simulink model "TCS_FrontAxle_Model"  (R2026a)
settings: Solver=ode4  StopTime=5  FixedStep=0.005
model workspace (MAT data in the model file):
  IntegralMax = 500
  IntegralMin = 0
  Ki = 200
  Kp = 800
  R_wheel = 0.25
  Tcorr_min_val = -500
  deadband = 0.02
  lambda_target = 0.1
  vx_min = 0.5
libraries: simulink x1
settings Model: Creator=liurui  LastModifiedBy=liurui

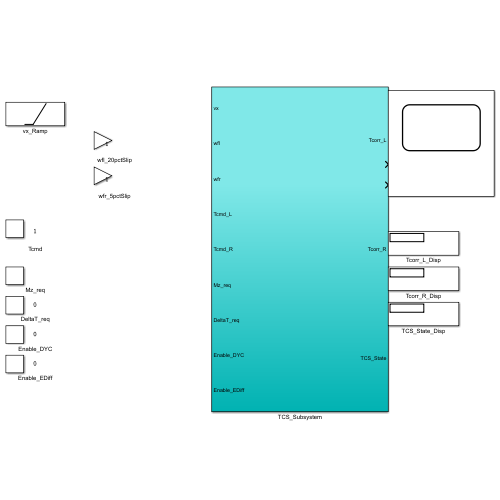
[thumbnail: Simulink's stored preview of the top-level diagram]
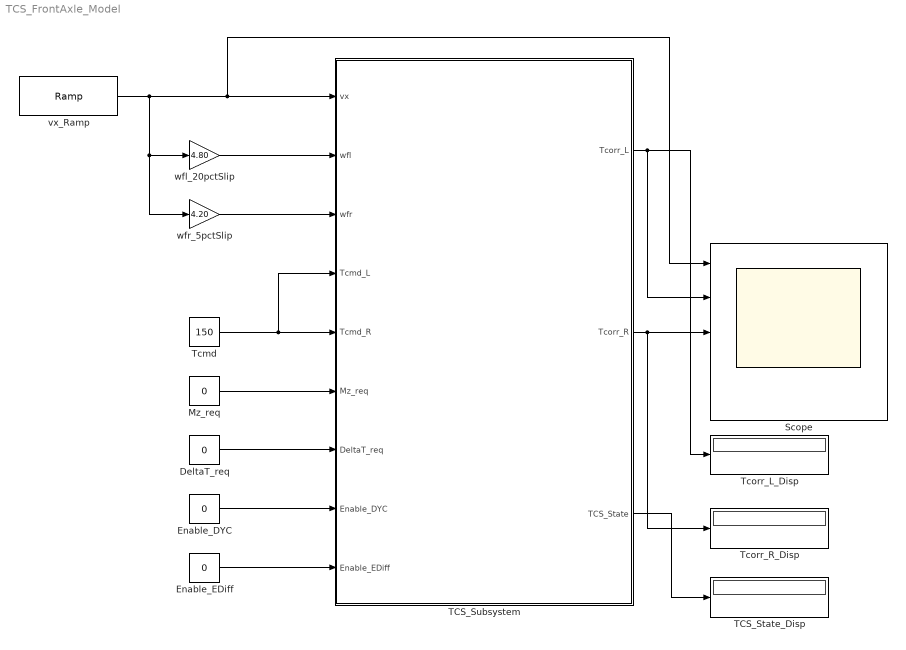
== system TCS_FrontAxle_Model ==
  DeltaT_req : Constant  Value=0
  Enable_DYC : Constant  Value=0
  Enable_EDiff : Constant  Value=0
  Mz_req : Constant  Value=0
  Scope : Scope  NumInputPorts=5
  TCS_State_Disp : Display
  TCS_Subsystem : Subsystem
  Tcmd : Constant  Value=150
  Tcorr_L_Disp : Display
  Tcorr_R_Disp : Display
  vx_Ramp : simulink/Sources/Ramp  slope=5  start=0.2  InitialOutput=0.1
  wfl_20pctSlip : Gain  Gain=4.80
  wfr_5pctSlip : Gain  Gain=4.20
  wires:
  vx_Ramp/1 -> wfl_20pctSlip/1, wfr_5pctSlip/1, TCS_Subsystem/1(vx), Scope/1
  Mz_req/1 -> TCS_Subsystem/6(Mz_req)
  Tcmd/1 -> TCS_Subsystem/4(Tcmd_L), TCS_Subsystem/5(Tcmd_R)
  wfr_5pctSlip/1 -> TCS_Subsystem/3(wfr)
  wfl_20pctSlip/1 -> TCS_Subsystem/2(wfl)
  Enable_EDiff/1 -> TCS_Subsystem/9(Enable_EDiff)
  Enable_DYC/1 -> TCS_Subsystem/8(Enable_DYC)
  TCS_Subsystem/2(Tcorr_R) -> Scope/3, Tcorr_R_Disp/1
  DeltaT_req/1 -> TCS_Subsystem/7(DeltaT_req)
  TCS_Subsystem/1(Tcorr_L) -> Scope/2, Tcorr_L_Disp/1
  TCS_Subsystem/3(TCS_State) -> TCS_State_Disp/1

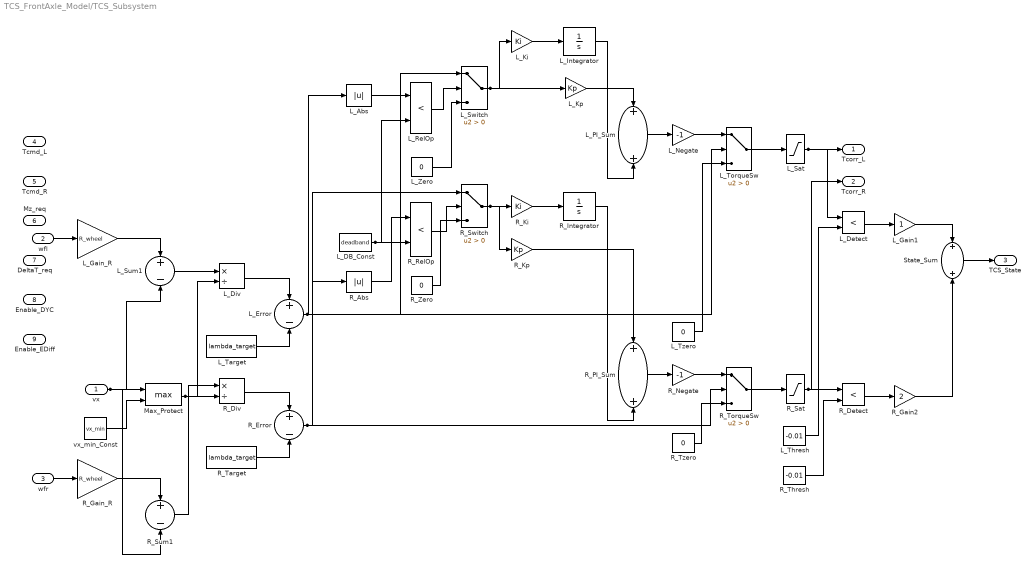
== system TCS_FrontAxle_Model/TCS_Subsystem ==
  vx : Inport
  wfl : Inport  Port=2
  wfr : Inport  Port=3
  Tcmd_L : Inport  Port=4
  Tcmd_R : Inport  Port=5
  Mz_req : Inport  Port=6
  DeltaT_req : Inport  Port=7
  Enable_DYC : Inport  Port=8
  Enable_EDiff : Inport  Port=9
  L_Abs : Abs  SaturateOnIntegerOverflow=off
  L_DB_Const : Constant  Value=deadband
  L_Detect : RelationalOperator  Operator=<  OutDataTypeStr=boolean  RndMeth=Simplest  InputSameDT=off
  L_Div : Product  Inputs=*/
  L_Error : Sum  Inputs=+-
  L_Gain1 : Gain
  L_Gain_R : Gain  Gain=R_wheel
  L_Integrator : Integrator  UpperSaturationLimit=IntegralMax  LowerSaturationLimit=IntegralMin
  L_Ki : Gain  Gain=Ki
  L_Kp : Gain  Gain=Kp
  L_Negate : Gain  Gain=-1
  L_PI_Sum : Sum
  L_RelOp : RelationalOperator  Operator=<  OutDataTypeStr=boolean  RndMeth=Simplest  InputSameDT=off
  L_Sat : Saturate  UpperLimit=0  LowerLimit=Tcorr_min_val
  L_Sum1 : Sum  Inputs=+-
  L_Switch : Switch  Criteria=u2 > Threshold  SaturateOnIntegerOverflow=off  InputSameDT=off
  L_Target : Constant  Value=lambda_target
  L_Thresh : Constant  Value=-0.01
  L_TorqueSw : Switch  Criteria=u2 > Threshold  SaturateOnIntegerOverflow=off  InputSameDT=off
  L_Tzero : Constant  Value=0
  L_Zero : Constant  Value=0
  Max_Protect : MinMax  Function=max  Inputs=2
  R_Abs : Abs  SaturateOnIntegerOverflow=off
  R_Detect : RelationalOperator  Operator=<  OutDataTypeStr=boolean  RndMeth=Simplest  InputSameDT=off
  R_Div : Product  Inputs=*/
  R_Error : Sum  Inputs=+-
  R_Gain2 : Gain  Gain=2
  R_Gain_R : Gain  Gain=R_wheel
  R_Integrator : Integrator  UpperSaturationLimit=IntegralMax  LowerSaturationLimit=IntegralMin
  R_Ki : Gain  Gain=Ki
  R_Kp : Gain  Gain=Kp
  R_Negate : Gain  Gain=-1
  R_PI_Sum : Sum
  R_RelOp : RelationalOperator  Operator=<  OutDataTypeStr=boolean  RndMeth=Simplest  InputSameDT=off
  R_Sat : Saturate  UpperLimit=0  LowerLimit=Tcorr_min_val
  R_Sum1 : Sum  Inputs=+-
  R_Switch : Switch  Criteria=u2 > Threshold  SaturateOnIntegerOverflow=off  InputSameDT=off
  R_Target : Constant  Value=lambda_target
  R_Thresh : Constant  Value=-0.01
  R_TorqueSw : Switch  Criteria=u2 > Threshold  SaturateOnIntegerOverflow=off  InputSameDT=off
  R_Tzero : Constant  Value=0
  R_Zero : Constant  Value=0
  State_Sum : Sum
  vx_min_Const : Constant  Value=vx_min
  Tcorr_L : Outport
  Tcorr_R : Outport  Port=2
  TCS_State : Outport  Port=3
  wires:
  wfr/1 -> R_Gain_R/1
  vx/1 -> R_Sum1/2, L_Sum1/2, Max_Protect/1
  wfl/1 -> L_Gain_R/1
  L_Ki/1 -> L_Integrator/1
  R_Switch/1 -> R_Kp/1, R_Ki/1
  L_Gain_R/1 -> L_Sum1/1
  vx_min_Const/1 -> Max_Protect/2
  Max_Protect/1 -> L_Div/2, R_Div/2
  R_Gain_R/1 -> R_Sum1/1
  L_Div/1 -> L_Error/1
  L_Sum1/1 -> L_Div/1
  R_Sum1/1 -> R_Div/1
  L_Negate/1 -> L_TorqueSw/1
  L_PI_Sum/1 -> L_Negate/1
  L_Target/1 -> L_Error/2
  R_Div/1 -> R_Error/1
  R_Target/1 -> R_Error/2
  L_Error/1 -> L_TorqueSw/2, L_Abs/1, L_Switch/1
  L_DB_Const/1 -> L_RelOp/2, R_RelOp/2
  R_Error/1 -> R_TorqueSw/2, R_Switch/1, R_Abs/1
  L_Abs/1 -> L_RelOp/1
  R_Abs/1 -> R_RelOp/1
  L_RelOp/1 -> L_Switch/2
  L_Zero/1 -> L_Switch/3
  R_RelOp/1 -> R_Switch/2
  R_Zero/1 -> R_Switch/3
  L_Switch/1 -> L_Kp/1, L_Ki/1
  R_Ki/1 -> R_Integrator/1
  R_Kp/1 -> R_PI_Sum/1
  L_Integrator/1 -> L_PI_Sum/2
  L_Kp/1 -> L_PI_Sum/1
  R_Integrator/1 -> R_PI_Sum/2
  L_TorqueSw/1 -> L_Sat/1
  R_PI_Sum/1 -> R_Negate/1
  L_Tzero/1 -> L_TorqueSw/3
  L_Thresh/1 -> L_Detect/2
  R_Negate/1 -> R_TorqueSw/1
  R_Tzero/1 -> R_TorqueSw/3
  L_Sat/1 -> L_Detect/1, Tcorr_L/1
  R_TorqueSw/1 -> R_Sat/1
  R_Sat/1 -> Tcorr_R/1, R_Detect/1
  L_Detect/1 -> L_Gain1/1
  R_Thresh/1 -> R_Detect/2
  R_Gain2/1 -> State_Sum/2
  R_Detect/1 -> R_Gain2/1
  L_Gain1/1 -> State_Sum/1
  State_Sum/1 -> TCS_State/1
